simulink model "Camera_Sensor_CS2017"  (R2014b)
settings: Solver=ode45  SolverMode=SingleTasking  StartTime=0  StopTime=40  FixedStep=0.001  RelTol=1e-3  AbsTol=1e-6
undefined symbols (not defined in the file): gray, strel
libraries: visionsinks x7, visionconversions x3, visiontextngfix x3, Solver_SF x2, visionanalysis x1, visionstatistics x1, visionmorphops x1
settings Model: CovSFcnEnable=on  ExtModeTrigMode=oneshot  ExtModeArmWhenConnect=off  Creator=ywata  LastModifiedBy=elowe
settings DataIOCC: LimitDataPoints=off  SignalLoggingSaveFormat=ModelDataLogs  SignalLoggingName=sigsOut
settings OptimizationCC: BlockReduction=off  BooleanDataType=off
settings DebuggingCC: SaveWithParameterizedLinksMsg=none  UnderspecifiedInitializationDetection=Classic  MergeDetectMultiDrivingBlocksExec=none  SignalResolutionControl=TryResolveAllWithWarning  SolverPrmCheckMsg=none  MultiTaskDSMMsg=warning  MultiTaskCondExecSysMsg=none  FcnCallInpInsideContextMsg=EnableAllAsWarning  FrameProcessingCompatibilityMsg=error  StateNameClashWarn=warning
settings HardwareCC: TargetUnknown=on
settings RTWCC: TemplateMakefile=grt_vc.tmf
settings GRTTargetCC: TargetFcnLib=ansi_tfl_tmw.mat  GeneratePreprocessorConditionals=Use local settings  CombineOutputUpdateFcns=off  GRTInterface=on

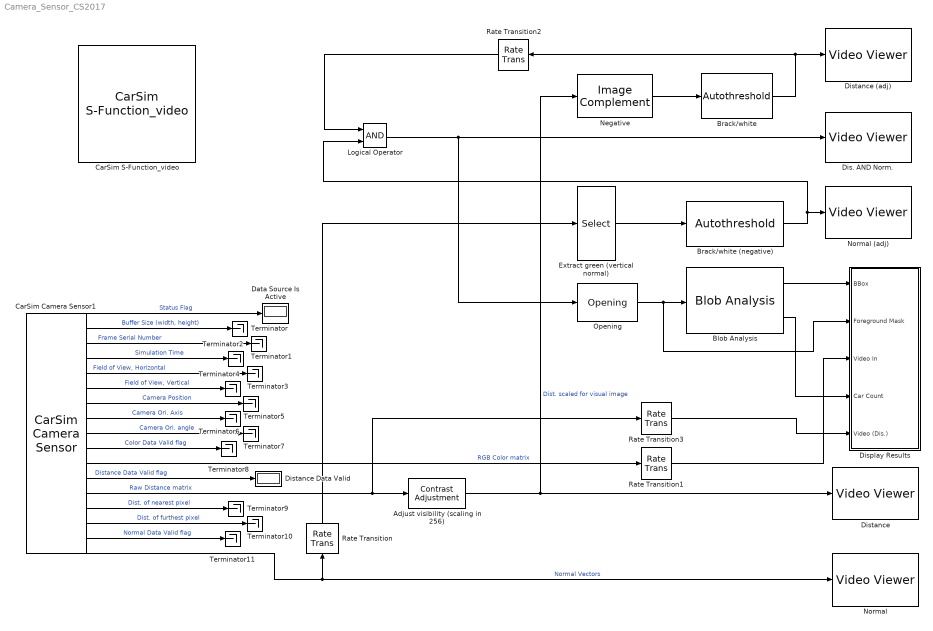
== system Camera_Sensor_CS2017 ==
  Adjust visibility (scaling in 256) : visionanalysis/Contrast Adjustment  methodInputRange=User-defined range  rangeIn=[0 256]  fracSaturate=[1 1]  isBinNum=on  binNum=256  methodOutputRange=Full data type range  rangeOut=[0 255]  prod1Mode=Binary point scaling  prod1WordLength=32  prod1FracLength=16  prod2Mode=Binary point scaling  prod2WordLength=32  prod2FracLength=16  roundingMode=Floor  overflowMode=off
  Blob Analysis : visionstatistics/Blob Analysis  Tag=vipblks_row_conv  area=off  centroid=off  bBox=on  majorAxis=off  minorAxis=off  angle=off  eccentricity=off  equivDiameterSq=off  extent=off  perimeter=off  maxBlobs=8  warnIfNumBlobsExceeded=on  isCount=on  useMinArea=on  minArea=150  useMaxArea=off  maxArea=intmax('uint32')  excludeBorderBlob=off  outDT=double  isOutVarDim=off  isFill=on  fillValues=-1  conn=8  isLabel=off  outputMode=Binary point scaling  outputWordLength=32  outputFracLength=16  firstCoeffMode=Binary point scaling  firstCoeffWordLength=16  firstCoeffFracLength=14  secondCoeffMode=Binary point scaling  secondCoeffWordLength=32  secondCoeffFracLength=16  accumMode=Binary point scaling  accumWordLength=32  accumFracLength=0  prodOutputMode=Binary point scaling  prodOutputWordLength=32  prodOutputFracLength=16  roundingMode=Floor  overflowMode=off
  Brack/white : visionconversions/Autothreshold  operator=>  threshOut=off  effMetricOut=off  userDefinedRange=off  umin=0  umax=255  outOfRngOpt=Warn and saturate  scaleThreshold=off  scaleFactor=1  P1Mode=Specify word length  P1WordLength=32  P1FracLength=30  P2Mode=Specify word length  P2WordLength=32  P2FracLength=22  P3Mode=Specify word length  P3WordLength=32  P3FracLength=14  P4Mode=Binary point scaling  P4WordLength=32  P4FracLength=15  Q1Mode=Specify word length  Q1WordLength=32  Q1FracLength=16  EMMode=Specify word length  EMWordLength=16  EMFracLength=14  roundingMode=Floor  overflowMode=off
  Brack/white (negative) : visionconversions/Autothreshold  operator=<=  threshOut=off  effMetricOut=off  userDefinedRange=off  umin=0  umax=255  outOfRngOpt=Warn and saturate  scaleThreshold=off  scaleFactor=1  P1Mode=Specify word length  P1WordLength=32  P1FracLength=30  P2Mode=Specify word length  P2WordLength=32  P2FracLength=22  P3Mode=Specify word length  P3WordLength=32  P3FracLength=14  P4Mode=Binary point scaling  P4WordLength=32  P4FracLength=15  Q1Mode=Specify word length  Q1WordLength=32  Q1FracLength=16  EMMode=Specify word length  EMWordLength=16  EMFracLength=14  roundingMode=Floor  overflowMode=off
  CarSim Camera Sensor1 : Solver_SF/CarSim Camera Sensor  Priority=1
  CarSim S-Function_video : Solver_SF/CarSim S-Function_video  Priority=1  SIMFILE=simfile.sim
  Data Source Is Active : Display
  Dis. AND Norm. : visionsinks/Video Viewer  inputType=Obsolete7b  imagePorts=One multidimensional signal  useColorMap=off  colormapValue=gray(256)  specRange=off  minInputVal=0  maxInputVal=255  FigPos=[805 1146 320 250]  AxisZoom=on  trueSizedOnce=off  OpenAtMdlStart=on  DefaultConfigurationName=vipscopes.VideoViewerScopeCfg
  Display Results : Subsystem
      settings: RTWMemSecFuncInitTerm=Default  RTWMemSecFuncExecute=Default  RTWMemSecDataConstants=Default  RTWMemSecDataInternal=Default  RTWMemSecDataParameters=Default
  Distance : visionsinks/Video Viewer  inputType=Obsolete7b  imagePorts=One multidimensional signal  useColorMap=off  colormapValue=gray(256)  specRange=off  minInputVal=0  maxInputVal=255  FigPos=[1451 352 320 259]  AxisZoom=on  trueSizedOnce=off  OpenAtMdlStart=on  DefaultConfigurationName=vipscopes.VideoViewerScopeCfg
  Distance (adj) : visionsinks/Video Viewer  inputType=Obsolete7b  imagePorts=One multidimensional signal  useColorMap=off  colormapValue=gray(256)  specRange=off  minInputVal=0  maxInputVal=255  FigPos=[1451 701 322 264]  AxisZoom=on  trueSizedOnce=off  OpenAtMdlStart=on  DefaultConfigurationName=vipscopes.VideoViewerScopeCfg
  Distance Data Valid : Display
  Extract green (vertical normal) : Selector  NumberOfDimensions=3  InputPortWidth=3  IndexOptions=Select all,Select all,Index vector (dialog)  Indices=(51:150),(51:270),2  OutputSizes=,1,1
  Logical Operator : Logic  AllPortsSameDT=off  OutDataTypeStr=boolean
  Negative : visionconversions/Image Complement
  Normal : visionsinks/Video Viewer  inputType=Obsolete7b  imagePorts=One multidimensional signal  useColorMap=off  colormapValue=gray(256)  specRange=off  minInputVal=0  maxInputVal=255  FigPos=[1449 1034 320 248]  AxisZoom=on  trueSizedOnce=off  OpenAtMdlStart=on  DefaultConfigurationName=vipscopes.VideoViewerScopeCfg
  Normal (adj) : visionsinks/Video Viewer  inputType=Obsolete7b  imagePorts=One multidimensional signal  useColorMap=off  colormapValue=gray(256)  specRange=off  minInputVal=0  maxInputVal=255  FigPos=[1126 1146 320 250]  AxisZoom=on  trueSizedOnce=off  OpenAtMdlStart=on  DefaultConfigurationName=vipscopes.VideoViewerScopeCfg
  Opening : visionmorphops/Opening  nhoodsrc=Specify via dialog  strel=strel('square', 4)
  Rate Transition{,1..3} (4 alike) : RateTransition  OutPortSampleTime=0.033
  Terminator{,1..11} (12 alike) : Terminator
  wires:
  CarSim Camera Sensor1/11 -> Rate Transition1/1  "RGB Color matrix"
  CarSim Camera Sensor1/1 -> Data Source Is Active/1  "Status Flag"
  Adjust visibility (scaling in 256)/1 -> Distance/1, Negative/1  "Dist. scaled for visual image"
  CarSim Camera Sensor1/13 -> Rate Transition3/1, Adjust visibility (scaling in 256)/1  "Raw Distance matrix"
  CarSim Camera Sensor1/17 -> Normal/1, Rate Transition/1  "Normal Vectors"
  CarSim Camera Sensor1/2 -> Terminator/1  "Buffer Size (width, height)"
  CarSim Camera Sensor1/14 -> Terminator9/1  "Dist. of nearest pixel"
  CarSim Camera Sensor1/15 -> Terminator10/1  "Dist. of furthest pixel"
  CarSim Camera Sensor1/16 -> Terminator11/1  "Normal Data Valid flag"
  CarSim Camera Sensor1/12 -> Distance Data Valid/1  "Distance Data Valid flag"
  CarSim Camera Sensor1/10 -> Terminator8/1  "Color Data Valid flag"
  CarSim Camera Sensor1/3 -> Terminator1/1  "Frame Serial Number"
  CarSim Camera Sensor1/4 -> Terminator2/1  "Simulation Time"
  CarSim Camera Sensor1/5 -> Terminator3/1  "Field of View, Horizontal"
  CarSim Camera Sensor1/6 -> Terminator4/1  "Field of View, Vertical"
  CarSim Camera Sensor1/7 -> Terminator5/1  "Camera Position"
  CarSim Camera Sensor1/8 -> Terminator6/1  "Camera Ori. Axis"
  CarSim Camera Sensor1/9 -> Terminator7/1  "Camera Ori. angle"
  Blob Analysis/1 -> Display Results/1(BBox)
  Rate Transition/1 -> Extract green (vertical normal)/1
  Rate Transition1/1 -> Display Results/3(Video In)
  Negative/1 -> Brack/white/1
  Extract green (vertical normal)/1 -> Brack/white (negative)/1
  Brack/white (negative)/1 -> Normal (adj)/1, Logical Operator/2
  Brack/white/1 -> Rate Transition2/1, Distance (adj)/1
  Opening/1 -> Blob Analysis/1, Display Results/2(Foreground Mask)
  Rate Transition2/1 -> Logical Operator/1
  Logical Operator/1 -> Opening/1, Dis. AND Norm./1
  Blob Analysis/2 -> Display Results/4(Car Count)
  Rate Transition3/1 -> Display Results/5(Video (Dis.))

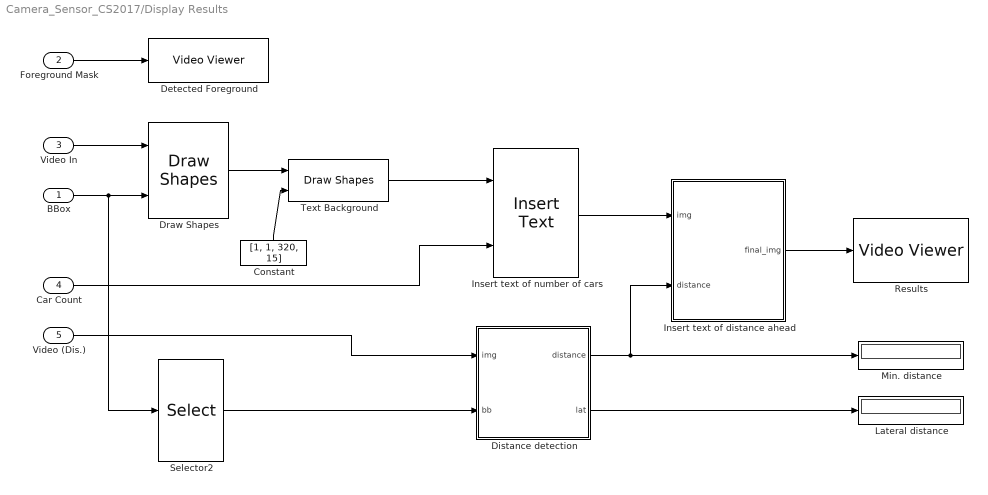
== system Camera_Sensor_CS2017/Display Results ==
  BBox : Inport
  Foreground Mask : Inport  Port=2
  Video In : Inport  Port=3
  Car Count : Inport  Port=4
  Video (Dis.) : Inport  Port=5
  Constant : Constant  Value=[1, 1, 320, 15]  OutDataTypeStr=uint32
  Detected Foreground : visionsinks/Video Viewer  inputType=Obsolete7b  imagePorts=One multidimensional signal  useColorMap=off  colormapValue=gray(256)  specRange=off  minInputVal=0  maxInputVal=255  FigPos=[467 1146 337 249]  AxisZoom=on  trueSizedOnce=on  OpenAtMdlStart=on  DefaultConfigurationName=vipscopes.VideoViewerScopeCfg
  Distance detection : MATLAB Function  TreatAsAtomicUnit=on
  Draw Shapes : visiontextngfix/Draw Shapes  shape=Rectangles  fill=off  lineWidth=1  fillClrSource=Specify via dialog  display=User-specified value  intensity=200  color=[0 256 0]  opacity=0.6  viewport=Entire image  antialiasing=off  inType=Obsolete  imagePorts=One multidimensional signal  prodOutputMode=Binary point scaling  prodOutputWordLength=32  prodOutputFracLength=14  memoryMode=Specify word length  memoryWordLength=16  memoryFracLength=15  roundingMode=Floor  overflowMode=off
  "Insert text of distance ahead " : MATLAB Function  TreatAsAtomicUnit=on
  Insert text of number of cars : visiontextngfix/Insert Text  inputType=Obsolete  theText='Number of Cars: %d'  getTextLocFrom=Specify via dialog  textLoc=[1 1]  getTextColorFrom=Specify via dialog  textColor=[256 256 256]  getTextIntensityFrom=Specify via dialog  textIntensity=1  getTextOpacityFrom=Specify via dialog  textOpacity=1.0  dummyVar2=0  dummyVar3=0  dummyVar4=0  imagePorts=One multidimensional signal  isInputTransposed=off  fontFace=LucidaTypewriterRegular  dummyVar1=0  blockFontSize=12  antiAliased=on
  Lateral distance : Display
  Min. distance : Display
  Results : visionsinks/Video Viewer  inputType=Obsolete7b  imagePorts=One multidimensional signal  useColorMap=off  colormapValue=gray(256)  specRange=off  minInputVal=0  maxInputVal=255  FigPos=[1 484 612 401]  AxisZoom=on  trueSizedOnce=on  OpenAtMdlStart=on  DefaultConfigurationName=vipscopes.VideoViewerScopeCfg
  Selector2 : Selector  NumberOfDimensions=2  InputPortWidth=3  IndexOptions=Select all,Select all  Indices=1,1  OutputSizes=99,1
  Text Background : visiontextngfix/Draw Shapes  shape=Rectangles  fill=on  lineWidth=1  fillClrSource=Specify via dialog  display=User-specified value  intensity=200  color=[0 0 0]  opacity=1  viewport=Entire image  antialiasing=off  inType=Obsolete  imagePorts=One multidimensional signal  prodOutputMode=Binary point scaling  prodOutputWordLength=32  prodOutputFracLength=14  memoryMode=Specify word length  memoryWordLength=16  memoryFracLength=14  roundingMode=Floor  overflowMode=off
  wires:
  Foreground Mask/1 -> Detected Foreground/1
  Text Background/1 -> Insert text of number of cars/1
  Video In/1 -> Draw Shapes/1
  Draw Shapes/1 -> Text Background/1
  Constant/1 -> Text Background/2
  Car Count/1 -> Insert text of number of cars/2
  BBox/1 -> Selector2/1, Draw Shapes/2
  Selector2/1 -> Distance detection/2(bb)
  Video (Dis.)/1 -> Distance detection/1(img)
  Distance detection/2(lat) -> Lateral distance/1
  Distance detection/1(distance) -> "Insert text of distance ahead "/2(distance), Min. distance/1
  Insert text of number of cars/1 -> "Insert text of distance ahead "/1(img)
  "Insert text of distance ahead "/1(final_img) -> Results/1

== matlab function Camera_Sensor_CS2017/Display Results/Distance detection ==
  data: img input; distance output; bb input; lat output
function [distance,lat] = fcn(img,bb)

angle_to_vehicle = 90.0;
lat_on_pixel = 0.0;

value_1_mem = 100.0;
value_2_mem = 100.0;

for i = 1:8
    if bb(i,1) < 0 
        value_1 = 100.0;
        value_2 = 100.0;
    else
        y = min(bb(i,2)+bb(i,4),200);
        x = min(bb(i,1)+bb(i,3),320);
        lat_on_pixel = double(bb(i,1)+bb(i,3)/2-160);
        angle_to_vehicle = double(lat_on_pixel/160*27.5);
    
        temp = img([bb(i,2):y],[bb(i,1):x]); 
        value_1 = double(min(temp(:)));
        value_2 = abs(value_1*tan(angle_to_vehicle/180*pi));
        
    end
    
    if value_2 < 1.3
        value_1_mem = value_1;
        value_2_mem = value_2;
    end
end

distance = value_1_mem;
lat = value_2_mem;

== matlab function Camera_Sensor_CS2017/Display Results/Insert text of distance ahead  ==
  data: img input; distance input; final_img output
function final_img = fcn(img, distance)

final_img = img;

coder.extrinsic('num2str');
coder.extrinsic('insertText');

dist = num2str(distance, '%0.1f');
if distance == 100
    dist = '> 100';
end
text = ['Distance Ahead: ' dist ' m'];

position = [160 8];

final_img = insertText(img,position,text, 'FontSize', 12, 'BoxColor',...
    'black', 'TextColor', 'white', 'BoxOpacity',0, 'AnchorPoint', 'LeftCenter');
